simulink model "VehicleFollowing"  (R2020a)
settings: Solver=VariableStepAuto  StartTime=0.0  StopTime=30  RelTol=1e-3
InitFcn:
  | load("bus.mat");
model workspace (MAT data in the model file):
  Acc_command : Simulink.Parameter (value not decoded)
  AngIn_command : Simulink.Parameter (value not decoded)
  Dece_command : Simulink.Parameter (value not decoded)
libraries: autolibutils x4, autolibshared x3, simulink x3, drivinglib x2, drivingscenarioandsensors x2, vrlib x2, vehdynlibsteering x1, mpcadaslib x1, robotalgslib x1
(part 3 of 3)

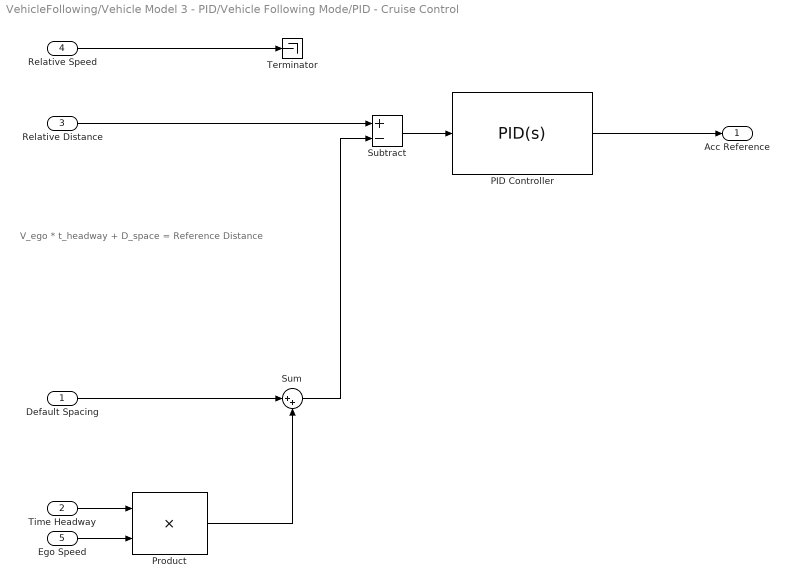
== system VehicleFollowing/Vehicle Model 3 - PID/Vehicle Following Mode/PID - Cruise Control ==
  note: V_ego * t_headway + D_space = Reference Distance
  Default Spacing : Inport
  Time Headway : Inport  Port=2
  Relative Distance : Inport  Port=3
  Relative Speed : Inport  Port=4
  Ego Speed : Inport  Port=5
  PID Controller : simulink/Continuous/PID Controller  Controller=PID  Form=Parallel  TimeDomain=Continuous-time  UseExternalTs=off  SampleTime=-1  IntegratorMethod=Forward Euler  FilterMethod=Forward Euler  ControllerParametersSource=internal  P=2  I=0.04  D=2.1  UseFilter=on  N=230  TunerSelectOption=Transfer Function Based (PID Tuner App)  InitialConditionSource=internal  InitialConditionForIntegrator=0  InitialConditionForFilter=0  DifferentiatorICPrevScaledInput=0  ExternalReset=none  TrackingMode=off  Kt=1  LimitOutput=on  UpperSaturationLimit=2  LowerSaturationLimit=-3  LinearizeAsGain=on  AntiWindupMode=clamping  Kb=1  POutMin=[]  POutMax=[]  IOutMin=[]  IOutMax=[]  DOutMin=[]  DOutMax=[]  NOutMin=[]  NOutMax=[]  SumOutMin=[]  SumOutMax=[]  SaturationOutMin=[]  SaturationOutMax=[]  PParamMin=[]  PParamMax=[]  IParamMin=[]  IParamMax=[]  DParamMin=[]  DParamMax=[]  NParamMin=[]  NParamMax=[]  KbParamMin=[]  KbParamMax=[]  KtParamMin=[]  KtParamMax=[]  KbOutMin=[]  KbOutMax=[]  KtOutMin=[]  KtOutMax=[]  IntegratorOutMin=[]  IntegratorOutMax=[]  FilterOutMin=[]  FilterOutMax=[]  SumI1OutMin=[]  SumI1OutMax=[]  SumI2OutMin=[]  SumI2OutMax=[]  SumI3OutMin=[]  SumI3OutMax=[]  SumI4OutMin=[]  SumI4OutMax=[]  SumDOutMin=[]  SumDOutMax=[]  DifferentiatorOutMin=[]  DifferentiatorOutMax=[]  FilterDiffOutCoefMin=[]  FilterDiffOutCoefMax=[]  ReciprocalOutMin=[]  ReciprocalOutMax=[]  SumDenOutMin=[]  SumDenOutMax=[]  SumNumOutMin=[]  SumNumOutMax=[]  DivideOutMin=[]  DivideOutMax=[]  UdiffTsProdOutMin=[]  UdiffTsProdOutMax=[]  NTsProdOutMin=[]  NTsProdOutMax=[]  UintegralTsProdOutMin=[]  UintegralTsProdOutMax=[]  UngainTsProdOutMin=[]  UngainTsProdOutMax=[]  IntegratorContinuousStateAttributes=''  IntegratorStateMustResolveToSignalObject=off  IntegratorRTWStateStorageClass=Auto  FilterContinuousStateAttributes=''  FilterStateMustResolveToSignalObject=off  FilterRTWStateStorageClass=Auto  ParallelPVariant=InternalParameters  IdealPVariant=Disabled  IVariant=InternalParameters  DVariant=InternalParameters  IntegratorVariant=Continuous  SatVariant=Enabled  AWVariant=ContClampingParallel  PCopyVariant=Disabled  TRVariant=Disabled  FdbkBlocksVariant=Forward  IdealPFdbkVariant=Disabled  SatFdbkVariant=Disabled  DerivativeFilterVariant=ContFilter  NVariant=InternalParameters  NCopyVariant=Disabled  FilterICVariant=InternalICsFilter  IntegratorICVariant=InternalICs  ExternalResetVariant=Disabled  TRSumVariant=Passthrough  SumFdbkVariant=Disabled  SumVariant=Sum_PID  TsampFilterVariant=InternalTs  TsampNgainVariant=Passthrough  TsampIntegralVariant=Passthrough
  Product : Product
  Subtract : Sum  Inputs=+-
  Sum : Sum  Inputs=|++
  Terminator : Terminator
  Acc Reference : Outport
  wires:
  Ego Speed/1 -> Product/2
  Time Headway/1 -> Product/1
  Default Spacing/1 -> Sum/1
  Product/1 -> Sum/2
  Sum/1 -> Subtract/2
  Relative Distance/1 -> Subtract/1
  Subtract/1 -> PID Controller/1
  PID Controller/1 -> Acc Reference/1
  Relative Speed/1 -> Terminator/1

== system VehicleFollowing/Vehicle Model 1 - Manual/Powertrain & Driveline/Driveline/AWD ==
  TPowertrain : Inport
  Gear : Inport  Port=2
  AWD : Gain  Gain=[1;1;1;1]./2
  Add : Sum
  Constant : Constant
  Constant1 : Constant  Value=zeros(4,1)
  Multiport Switch : MultiPortSwitch  DataPortOrder=Zero-based contiguous  zeroidx=on
  Unary Minus : UnaryMinus
  TAxles : Outport  VectorParamsAs1DForOutWhenUnconnected=off
  wires:
  TPowertrain/1 -> AWD/1
  Multiport Switch/1 -> TAxles/1
  Add/1 -> Multiport Switch/1
  Constant1/1 -> Multiport Switch/3
  AWD/1 -> Unary Minus/1, Multiport Switch/4
  Constant/1 -> Add/2
  Gear/1 -> Add/1
  Unary Minus/1 -> Multiport Switch/2

== system VehicleFollowing/Vehicle Model 1 - Manual/Powertrain & Driveline/Driveline/FWD ==
  TPowertrain : Inport
  Gear : Inport  Port=2
  Add : Sum
  Constant : Constant
  Constant1 : Constant  Value=zeros(4,1)
  FWD : Gain  Gain=[1;1;0;0]
  Multiport Switch : MultiPortSwitch  DataPortOrder=Zero-based contiguous  zeroidx=on
  Unary Minus : UnaryMinus
  TAxles : Outport  VectorParamsAs1DForOutWhenUnconnected=off
  wires:
  TPowertrain/1 -> FWD/1
  Multiport Switch/1 -> TAxles/1
  Add/1 -> Multiport Switch/1
  Constant1/1 -> Multiport Switch/3
  FWD/1 -> Unary Minus/1, Multiport Switch/4
  Constant/1 -> Add/2
  Gear/1 -> Add/1
  Unary Minus/1 -> Multiport Switch/2

== system VehicleFollowing/Vehicle Model 1 - Manual/Powertrain & Driveline/Driveline/RWD ==
  TPowertrain : Inport
  Gear : Inport  Port=2
  Add : Sum
  Constant : Constant
  Constant1 : Constant  Value=zeros(4,1)
  Multiport Switch : MultiPortSwitch  DataPortOrder=Zero-based contiguous  zeroidx=on
  RWD : Gain  Gain=[0;0;1;1]
  Unary Minus : UnaryMinus
  TAxles : Outport  VectorParamsAs1DForOutWhenUnconnected=off
  wires:
  RWD/1 -> Unary Minus/1, Multiport Switch/4
  TPowertrain/1 -> RWD/1
  Unary Minus/1 -> Multiport Switch/2
  Multiport Switch/1 -> TAxles/1
  Gear/1 -> Add/1
  Constant/1 -> Add/2
  Add/1 -> Multiport Switch/1
  Constant1/1 -> Multiport Switch/3

== stateflow chart VehicleFollowing/Vehicle Model 3 - PID/Driving Mode Selector ==
  state FreeDrive
    entry:
    driving_mode=0;
  state LeftSwitch
    entry:
    driving_mode=4;
  state Wait
    entry:
    driving_mode=0
  (default) -> FreeDrive
  FreeDrive -> LeftSwitch : [command==0x01]
  LeftSwitch -> Wait : [after(0.4,sec)]
  Wait -> FreeDrive : [lane_switch_finish==1]
  data: command input; lane_switch_finish input; driving_mode output

== matlab function VehicleFollowing/2D Animation/MATLAB Function ==
  data: V1_Pose input; V2_Pose input; V3_Pose input
function plotVehicle(V1_Pose, V2_Pose, V3_Pose)
%% Prepare the trace of Vehicle 3 % Uncomment this section + the "plot" function for Vehicle 3's trace
% persistent x_old y_old 
% 
% if isempty(x_old)
%     x_old = V3_Pose(1);
% else
%     x_old = [x_old V3_Pose(1)];
% end
% 
% if isempty(y_old)
%     y_old = V3_Pose(2);
% else
%     y_old = [y_old V3_Pose(2)];
% end
%% Clear previous Vehicle
cla;

%% Vehicle 1 - Pose
x1 = V1_Pose(1);
y1 = V1_Pose(2);
yaw1 = V1_Pose(3);

centerP = [x1;y1];

V1_HalfLength = 2; % Length = 4m
V1_HalfWidth = 1; % Width = 2m

% Creating a rectangle
p1 = [V1_HalfLength; V1_HalfWidth];
p2 = [V1_HalfLength; -V1_HalfWidth];
p3 = [-V1_HalfLength; -V1_HalfWidth];
p4 = [-V1_HalfLength; V1_HalfWidth];

% Rotation Matrix
Rmatrix = [cos(yaw1) -sin(yaw1); sin(yaw1) cos(yaw1)];

% Rotated Points
p1r = centerP + Rmatrix*p1;
p2r = centerP + Rmatrix*p2;
p3r = centerP + Rmatrix*p3;
p4r = centerP + Rmatrix*p4;

% Connecting points
Hitbox_V1 = [p1r p2r p3r p4r p1r];

cornersV1_x = transpose(Hitbox_V1(1,:));
cornersV1_y = transpose(Hitbox_V1(2,:));

%% Vehicle 2 - Pose
x2 = V2_Pose(1);
y2 = V2_Pose(2);
yaw2 = V2_Pose(3);

centerP = [x2;y2];

V2_HalfLength = 2; % Length = 4m
V2_HalfWidth = 1; % Width = 2m

% Creating a rectangle
p1 = [V2_HalfLength; V2_HalfWidth];
p2 = [V2_HalfLength; -V2_HalfWidth];
p3 = [-V2_HalfLength; -V2_HalfWidth];
p4 = [-V2_HalfLength; V2_HalfWidth];

% Rotation Matrix

Rmatrix = [cos(yaw2) -sin(yaw2); sin(yaw2) cos(yaw2)];

% Rotated Points
p1r = centerP + Rmatrix*p1;
p2r = centerP + Rmatrix*p2;
p3r = centerP + Rmatrix*p3;
p4r = centerP + Rmatrix*p4;

% Connecting points
Hitbox_V2 = [p1r p2r p3r p4r p1r];

cornersV2_x = transpose(Hitbox_V2(1,:));
cornersV2_y = transpose(Hitbox_V2(2,:));

%% Vehicle 3 - Pose
x3 = V3_Pose(1);
y3 = V3_Pose(2);
yaw3 = V3_Pose(3);

centerP = [x3;y3];

V3_HalfLength = 2; % Length = 4m
V3_HalfWidth = 1; % Width = 2m

% Creating a rectangle
p1 = [V3_HalfLength; V3_HalfWidth];
p2 = [V3_HalfLength; -V3_HalfWidth];
p3 = [-V3_HalfLength; -V3_HalfWidth];
p4 = [-V3_HalfLength; V3_HalfWidth];

% Rotation Matrix
Rmatrix = [cos(yaw3) -sin(yaw3); sin(yaw3) cos(yaw3)];

% Rotated Points
p1r = centerP + Rmatrix*p1;
p2r = centerP + Rmatrix*p2;
p3r = centerP + Rmatrix*p3;
p4r = centerP + Rmatrix*p4;

% Connecting points
Hitbox_V3 = [p1r p2r p3r p4r p1r];

cornersV3_x = transpose(Hitbox_V3(1,:));
cornersV3_y = transpose(Hitbox_V3(2,:));

%% Plot Vehicles and the road
plot(cornersV1_x,cornersV1_y,'g'); %Vehicle 1 rectangle
plot(x1,y1,'*'); %Vehicle 1 center

plot(cornersV2_x,cornersV2_y,'r'); %Vehicle 2 rectangle
plot(x2,y2,'o'); %Vehicle 2 center

plot(cornersV3_x,cornersV3_y,'b'); %Vehicle 3 rectangle
plot(x3,y3,'x'); %Vehicle 3 center
%plot(x_old,y_old,'x'); % To plot the trace of Vehicle 3

upperLine = plot([0 1000], [5 5], 'Color', 'blue');
midLine = plot([0 1000], [0 0],'--', 'Color', 'blue');
lowerLine = plot([0 1000], [-5 -5], 'Color', 'blue');




% Adjust Axis
axis([x3-200 x3+200 y3-20 y3+20]); % Camera following V3 as ego vehicle

== stateflow chart VehicleFollowing/Vehicle Model 2 - MPC/Driving Mode Selector ==
  state VehicleFollowing
    entry:
    drivingMode=2;
  state FreeDrive
    entry:
    drivingMode =1;
  state EmergecyBrake
    entry:
    drivingMode=3;
  (default) -> FreeDrive
  VehicleFollowing -> FreeDrive [order 1] : [relativeDistance >100]
  FreeDrive -> VehicleFollowing [order 1] : [relativeDistance <=95]
  FreeDrive -> EmergecyBrake [order 2] : [relativeDistance <=10]
  VehicleFollowing -> EmergecyBrake [order 2] : [relativeDistance <=10]
  EmergecyBrake -> VehicleFollowing : [relativeDistance>15]
  data: relativeDistance input; drivingMode output

== matlab function VehicleFollowing/2D Animation2/Pack Ego Actor ==
  data: pos input; egoActor output Bus: BusActors1Actors size=1; vel input; yaw input; yawRate input
function egoActor = packEgo(pos,vel,yaw,yawRate)
% Pack ego information into a single ego actor bus
%
% Imoprtant note:
% Output is a bus of type BusActorsActors. This is the same bus used by the
% Scenario Reader to output an individual actor. If you change the
% output bus name of Scenario Reader, change the output bus name here
% as well by clicking on 'Edit Data' in the menu above.
% if pos(2)<=-2
%     pos(2)=-2;
% elseif pos(2)>=2
%     pos(2)=2;
% end

egoActor = struct(...
    'ActorID',1,...
    'Position', [pos(1) pos(2) 0], ...
    'Velocity', [vel(1) vel(2) 0], ...
    'Roll', 0, ...
    'Pitch', 0, ...
    'Yaw', yaw, ...
    'AngularVelocity', [0 0 yawRate]);
